simulink model "task_simulation_wo_atan_wo_saturation"  (R2025b)
settings: Solver=VariableStepAuto  StartTime=0.0  StopTime=20  FixedStep=0.001  RelTol=1e-3
InitFcn:
  | prepare_parameters
undefined symbols (not defined in the file): I_max_val, J_1_val, J_2_val, k_E_val, k_M_val, k_t_val, L_val, R_val, U_max_val
libraries: simulink_extras x5, slpidlib x2, embmathops x1
settings Model: Creator=10120  LastModifiedBy=10120

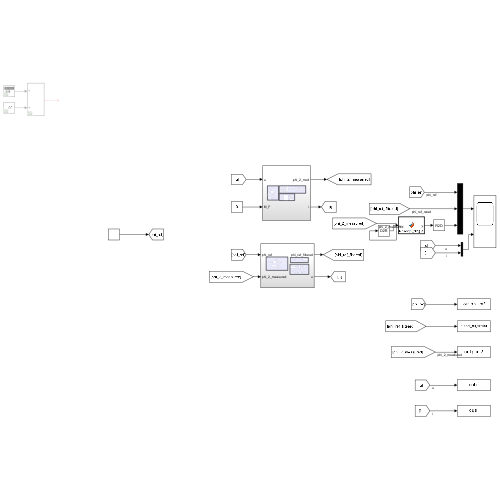
[thumbnail: Simulink's stored preview of the top-level diagram]
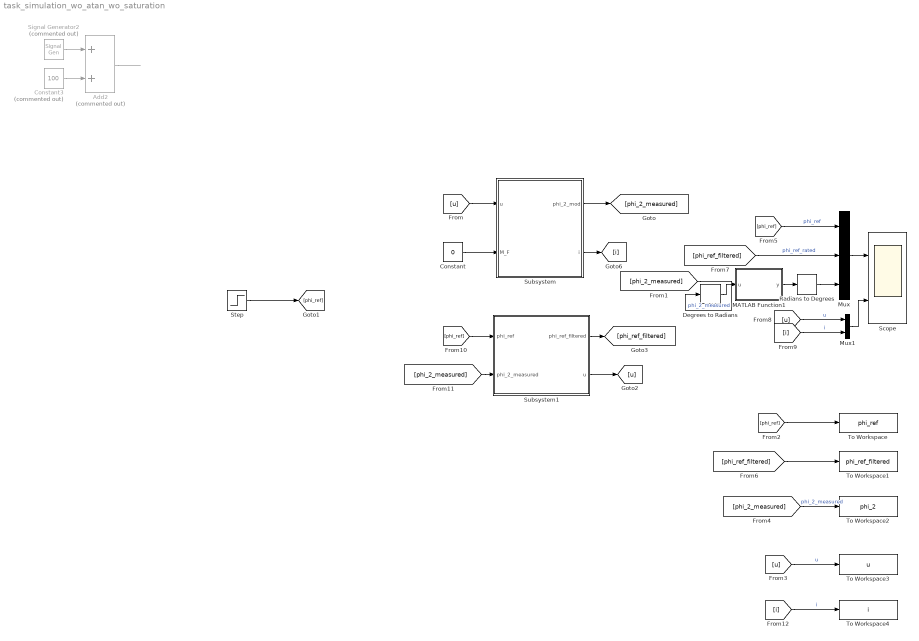
== system task_simulation_wo_atan_wo_saturation ==
  Add2 : Sum  Commented=on
  Constant : Constant  Value=0
  Constant3 : Constant  Commented=on  Value=100
  Degrees to Radians : simulink_extras/Transformations/Degrees to Radians
  MATLAB Function1 : MATLAB Function  TreatAsAtomicUnit=on
  Mux : Mux  Inputs=3
  Mux1 : Mux  Inputs=2
  Radians to Degrees : simulink_extras/Transformations/Radians to Degrees
  Scope : Scope  NumInputPorts=2
      settings: ActiveDisplayYMinimum=-44.999984027825569  ActiveDisplayYMaximum=404.99985625043018
  Signal Generator2 : SignalGenerator  Commented=on  Amplitude=100  Frequency=0.1  Units=rad/sec
  Step : Step  Time=0.1  After=200  SampleTime=0
  Subsystem : Subsystem
  Subsystem1 : Subsystem
  To Workspace : ToWorkspace  VariableName=phi_ref  SaveFormat=Structure With Time  SampleTime=-1
  To Workspace1 : ToWorkspace  VariableName=phi_ref_filtered  SaveFormat=Structure With Time  SampleTime=-1
  To Workspace2 : ToWorkspace  VariableName=phi_2  SaveFormat=Structure With Time  SampleTime=-1
  To Workspace3 : ToWorkspace  VariableName=u  SaveFormat=Structure With Time  SampleTime=-1
  To Workspace4 : ToWorkspace  VariableName=i  SaveFormat=Structure With Time  SampleTime=-1
  wires:
  Constant/1 -> Subsystem/2(M_F)
  [u] -> Subsystem/1(u)
  Subsystem/1(phi_2_mod) -> [phi_2_measured]
  Step/1 -> [phi_ref]
  Add2/1 -> ?
  Constant3/1 -> Add2/2
  Signal Generator2/1 -> Add2/1
  Mux/1 -> Scope/1
  [phi_ref] -> Mux/1  "phi_ref"
  [phi_ref_filtered] -> Mux/2  "phi_ref_rated"
  Subsystem/2(i) -> [i]
  [phi_ref] -> Subsystem1/1(phi_ref)
  [phi_2_measured] -> Subsystem1/2(phi_2_measured)
  Subsystem1/2(u) -> [u]
  Subsystem1/1(phi_ref_filtered) -> [phi_ref_filtered]
  Mux1/1 -> Scope/2
  [u] -> Mux1/1  "u"
  [i] -> Mux1/2  "i"
  [phi_ref] -> To Workspace/1
  [phi_ref_filtered] -> To Workspace1/1
  [phi_2_measured] -> To Workspace2/1  "phi_2_measured"
  [u] -> To Workspace3/1  "u"
  [i] -> To Workspace4/1  "i"
  Degrees to Radians/1 -> MATLAB Function1/1(u)
  MATLAB Function1/1(y) -> Radians to Degrees/1
  Radians to Degrees/1 -> Mux/3
  [phi_2_measured] -> Degrees to Radians/1  "phi_2_measured"

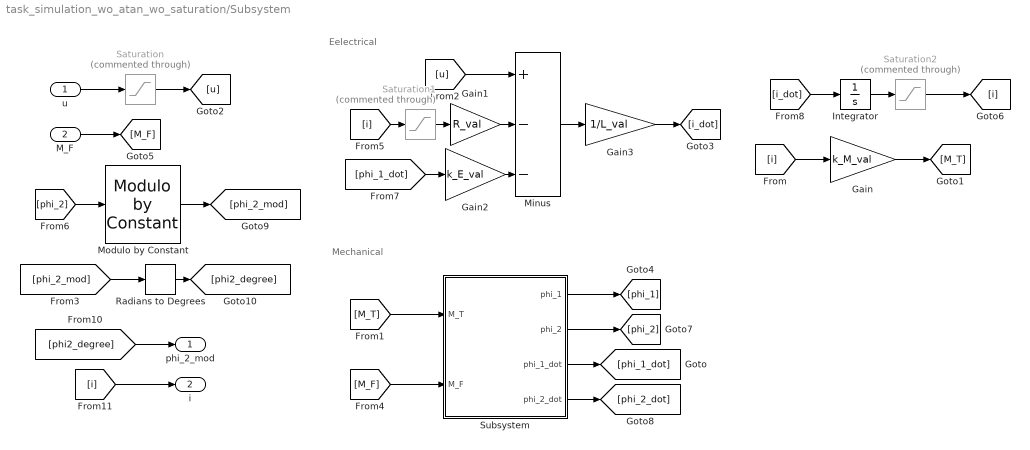
== system task_simulation_wo_atan_wo_saturation/Subsystem ==
  note: Mechanical
  note: Eelectrical
  u : Inport
  M_F : Inport  Port=2
  Gain : Gain  Gain=k_M_val
  Gain1 : Gain  Gain=R_val
  Gain2 : Gain  Gain=k_E_val
  Gain3 : Gain  Gain=1/L_val
  Integrator : Integrator
  Minus : Sum  Inputs=+--
  Modulo by Constant : embmathops/Modulo by Constant  Denominator=2*pi  SimulateUsing=Code generation
      settings: LibrarySourceBlock=embeddedMathLib/Modulo by Constant
  Radians to Degrees : simulink_extras/Transformations/Radians to Degrees
  Saturation : Saturate  Commented=through  UpperLimit=U_max_val  LowerLimit=-U_max_val
  Saturation1 : Saturate  Commented=through  UpperLimit=I_max_val  LowerLimit=-I_max_val
  Saturation2 : Saturate  Commented=through  UpperLimit=I_max_val  LowerLimit=-I_max_val
  Subsystem : Subsystem
  phi_2_mod : Outport
  i : Outport  Port=2
  wires:
  [i] -> Gain/1
  Gain/1 -> [M_T]
  [M_T] -> Subsystem/1(M_T)
  u/1 -> Saturation/1
  Gain3/1 -> [i_dot]
  [u] -> Minus/1
  Gain1/1 -> Minus/2
  [i] -> Saturation1/1
  Subsystem/1(phi_1) -> [phi_1]
  Gain2/1 -> Minus/3
  [phi_1_dot] -> Gain2/1
  Minus/1 -> Gain3/1
  [i_dot] -> Integrator/1
  Integrator/1 -> Saturation2/1
  Subsystem/3(phi_1_dot) -> [phi_1_dot]
  [phi2_degree] -> phi_2_mod/1
  M_F/1 -> [M_F]
  [M_F] -> Subsystem/2(M_F)
  Subsystem/2(phi_2) -> [phi_2]
  Subsystem/4(phi_2_dot) -> [phi_2_dot]
  [phi_2] -> Modulo by Constant/1
  Modulo by Constant/1 -> [phi_2_mod]
  Saturation/1 -> [u]
  Saturation1/1 -> Gain1/1
  Saturation2/1 -> [i]
  [i] -> i/1
  [phi_2_mod] -> Radians to Degrees/1
  Radians to Degrees/1 -> [phi2_degree]

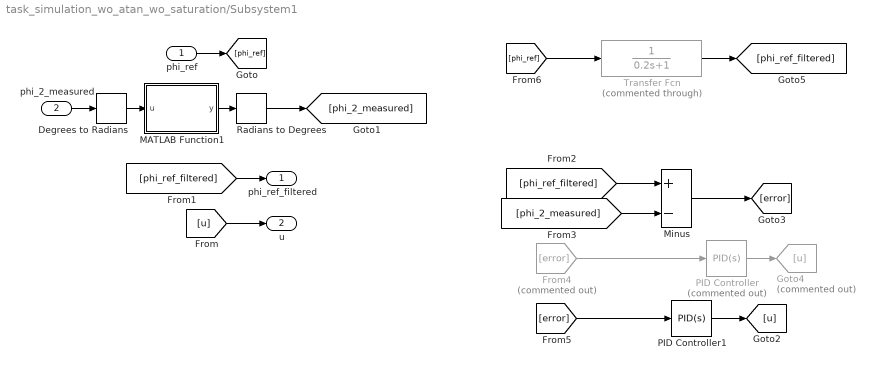
== system task_simulation_wo_atan_wo_saturation/Subsystem1 ==
  phi_ref : Inport
  phi_2_measured : Inport  Port=2
  Degrees to Radians : simulink_extras/Transformations/Degrees to Radians
  From4 : From  Commented=on  GotoTag=error
  Goto4 : Goto  Commented=on  GotoTag=u
  MATLAB Function1 : MATLAB Function  TreatAsAtomicUnit=on
  Minus : Sum  Inputs=+-
  PID Controller : slpidlib/PID Controller  Commented=on  Controller=PID  Form=Parallel  TimeDomain=Continuous-time  UseExternalTs=off  SampleTime=-1  IntegratorMethod=Forward Euler  FilterMethod=Forward Euler  ControllerParametersSource=internal  P=0.02  I=0  UseKiTs=off  D=0.5/360  UseExternalDerivativeSource=off  N=1  UseFilter=on  TunerSelectOption=Transfer Function Based (PID Tuner App)  InitialConditionSource=internal  InitialConditionForIntegrator=0  InitialConditionForFilter=0  DifferentiatorICPrevScaledInput=0  ExternalReset=none  TrackingMode=off  Kt=1  LimitOutput=on  SatLimitsSource=internal  UpperSaturationLimit=U_max_val  LowerSaturationLimit=-U_max_val  LinearizeAsGain=on  AntiWindupMode=clamping  Kb=1  LimitIntegrator=off  UpperIntegratorSaturationLimit=inf  LowerIntegratorSaturationLimit=-inf  POutMin=[]  POutMax=[]  IOutMin=[]  IOutMax=[]  DOutMin=[]  DOutMax=[]  NOutMin=[]  NOutMax=[]  SumOutMin=[]  SumOutMax=[]  SaturationOutMin=[]  SaturationOutMax=[]  PParamMin=[]  PParamMax=[]  IParamMin=[]  IParamMax=[]  DParamMin=[]  DParamMax=[]  NParamMin=[]  NParamMax=[]  KbParamMin=[]  KbParamMax=[]  KtParamMin=[]  KtParamMax=[]  KbOutMin=[]  KbOutMax=[]  KtOutMin=[]  KtOutMax=[]  IntegratorOutMin=[]  IntegratorOutMax=[]  FilterOutMin=[]  FilterOutMax=[]  SumI1OutMin=[]  SumI1OutMax=[]  SumI2OutMin=[]  SumI2OutMax=[]  SumI3OutMin=[]  SumI3OutMax=[]  SumI4OutMin=[]  SumI4OutMax=[]  SumDOutMin=[]  SumDOutMax=[]  DifferentiatorOutMin=[]  DifferentiatorOutMax=[]  FilterDiffOutCoefMin=[]  FilterDiffOutCoefMax=[]  ReciprocalOutMin=[]  ReciprocalOutMax=[]  SumDenOutMin=[]  SumDenOutMax=[]  SumNumOutMin=[]  SumNumOutMax=[]  DivideOutMin=[]  DivideOutMax=[]  UdiffTsProdOutMin=[]  UdiffTsProdOutMax=[]  NTsProdOutMin=[]  NTsProdOutMax=[]  UintegralTsProdOutMin=[]  UintegralTsProdOutMax=[]  UngainTsProdOutMin=[]  UngainTsProdOutMax=[]  ClampingZeroOutDataTypeStr=Inherit: Inherit via back propagation  ClampingZeroOutMin=[]  ClampingZeroOutMax=[]  FilterDenConstantOutDataTypeStr=Inherit: Inherit via back propagation  FilterDenConstantOutMin=[]  FilterDenConstantOutMax=[]  PCopyOutDataTypeStr=Inherit: Inherit via back propagation  PCopyOutMin=[]  PCopyOutMax=[]  NCopyOutDataTypeStr=Inherit: Inherit via back propagation  NCopyOutMin=[]  NCopyOutMax=[]  IntegratorContinuousStateAttributes=''  IntegratorStateMustResolveToSignalObject=off  IntegratorRTWStateStorageClass=Auto  FilterContinuousStateAttributes=''  FilterStateMustResolveToSignalObject=off  FilterRTWStateStorageClass=Auto  ParallelPVariant=InternalParameters  IdealPVariant=Disabled  IVariant=InternalParameters  DVariant=InternalParameters  IntegratorVariant=Continuous  SatVariant=Enabled  AWVariant=ContClampingParallel  PCopyVariant=Disabled  TRVariant=Disabled  FdbkBlocksVariant=Forward  IdealPFdbkVariant=Disabled  SatFdbkVariant=Disabled  DerivativeFilterVariant=ContFilter  NVariant=InternalParameters  NCopyVariant=Disabled  FilterICVariant=InternalICsFilter  IntegratorICVariant=InternalICs  ExternalResetVariant=Disabled  TRSumVariant=Passthrough  SumFdbkVariant=Disabled  SumVariant=Sum_PID  TsampFilterVariant=InternalTs  TsampNgainVariant=Passthrough  TsampIntegralVariant=Disabled_SignalSpec  ExternalSaturationOutDataTypeStr=Inherit: Same as second input  DerivativeSourceVariant=ErrorSignal  PreIntVariant=InternalPreInt
  PID Controller1 : slpidlib/PID Controller  Controller=PID  Form=Parallel  TimeDomain=Continuous-time  UseExternalTs=off  SampleTime=-1  IntegratorMethod=Forward Euler  FilterMethod=Forward Euler  ControllerParametersSource=internal  P=1  I=0  UseKiTs=off  D=0  UseExternalDerivativeSource=off  N=1  UseFilter=on  TunerSelectOption=Transfer Function Based (PID Tuner App)  InitialConditionSource=internal  InitialConditionForIntegrator=0  InitialConditionForFilter=0  DifferentiatorICPrevScaledInput=0  ExternalReset=none  TrackingMode=off  Kt=1  LimitOutput=off  SatLimitsSource=internal  UpperSaturationLimit=U_max_val  LowerSaturationLimit=-U_max_val  LinearizeAsGain=on  AntiWindupMode=clamping  Kb=1  LimitIntegrator=off  UpperIntegratorSaturationLimit=inf  LowerIntegratorSaturationLimit=-inf  POutMin=[]  POutMax=[]  IOutMin=[]  IOutMax=[]  DOutMin=[]  DOutMax=[]  NOutMin=[]  NOutMax=[]  SumOutMin=[]  SumOutMax=[]  SaturationOutMin=[]  SaturationOutMax=[]  PParamMin=[]  PParamMax=[]  IParamMin=[]  IParamMax=[]  DParamMin=[]  DParamMax=[]  NParamMin=[]  NParamMax=[]  KbParamMin=[]  KbParamMax=[]  KtParamMin=[]  KtParamMax=[]  KbOutMin=[]  KbOutMax=[]  KtOutMin=[]  KtOutMax=[]  IntegratorOutMin=[]  IntegratorOutMax=[]  FilterOutMin=[]  FilterOutMax=[]  SumI1OutMin=[]  SumI1OutMax=[]  SumI2OutMin=[]  SumI2OutMax=[]  SumI3OutMin=[]  SumI3OutMax=[]  SumI4OutMin=[]  SumI4OutMax=[]  SumDOutMin=[]  SumDOutMax=[]  DifferentiatorOutMin=[]  DifferentiatorOutMax=[]  FilterDiffOutCoefMin=[]  FilterDiffOutCoefMax=[]  ReciprocalOutMin=[]  ReciprocalOutMax=[]  SumDenOutMin=[]  SumDenOutMax=[]  SumNumOutMin=[]  SumNumOutMax=[]  DivideOutMin=[]  DivideOutMax=[]  UdiffTsProdOutMin=[]  UdiffTsProdOutMax=[]  NTsProdOutMin=[]  NTsProdOutMax=[]  UintegralTsProdOutMin=[]  UintegralTsProdOutMax=[]  UngainTsProdOutMin=[]  UngainTsProdOutMax=[]  ClampingZeroOutDataTypeStr=Inherit: Inherit via back propagation  ClampingZeroOutMin=[]  ClampingZeroOutMax=[]  FilterDenConstantOutDataTypeStr=Inherit: Inherit via back propagation  FilterDenConstantOutMin=[]  FilterDenConstantOutMax=[]  PCopyOutDataTypeStr=Inherit: Inherit via back propagation  PCopyOutMin=[]  PCopyOutMax=[]  NCopyOutDataTypeStr=Inherit: Inherit via back propagation  NCopyOutMin=[]  NCopyOutMax=[]  IntegratorContinuousStateAttributes=''  IntegratorStateMustResolveToSignalObject=off  IntegratorRTWStateStorageClass=Auto  FilterContinuousStateAttributes=''  FilterStateMustResolveToSignalObject=off  FilterRTWStateStorageClass=Auto  ParallelPVariant=InternalParameters  IdealPVariant=Disabled  IVariant=InternalParameters  DVariant=InternalParameters  IntegratorVariant=Continuous  SatVariant=Disabled  AWVariant=Passthrough  PCopyVariant=Disabled  TRVariant=Disabled  FdbkBlocksVariant=Forward  IdealPFdbkVariant=Disabled  SatFdbkVariant=Disabled  DerivativeFilterVariant=ContFilter  NVariant=InternalParameters  NCopyVariant=Disabled  FilterICVariant=InternalICsFilter  IntegratorICVariant=InternalICs  ExternalResetVariant=Disabled  TRSumVariant=Passthrough  SumFdbkVariant=Disabled  SumVariant=Sum_PID  TsampFilterVariant=InternalTs  TsampNgainVariant=Passthrough  TsampIntegralVariant=Disabled_SignalSpec  ExternalSaturationOutDataTypeStr=Inherit: Same as second input  DerivativeSourceVariant=ErrorSignal  PreIntVariant=InternalPreInt
  Radians to Degrees : simulink_extras/Transformations/Radians to Degrees
  Transfer Fcn : TransferFcn  Commented=through  Denominator=[0.2 1]
  phi_ref_filtered : Outport
  u : Outport  Port=2
  wires:
  Minus/1 -> [error]
  PID Controller/1 -> Goto4/1
  From4/1 -> PID Controller/1
  Transfer Fcn/1 -> [phi_ref_filtered]
  [phi_2_measured] -> Minus/2
  [phi_ref] -> Transfer Fcn/1
  [phi_ref_filtered] -> Minus/1
  phi_ref/1 -> [phi_ref]
  phi_2_measured/1 -> Degrees to Radians/1
  [phi_ref_filtered] -> phi_ref_filtered/1
  [u] -> u/1
  PID Controller1/1 -> [u]
  [error] -> PID Controller1/1
  Degrees to Radians/1 -> MATLAB Function1/1(u)
  MATLAB Function1/1(y) -> Radians to Degrees/1
  Radians to Degrees/1 -> [phi_2_measured]

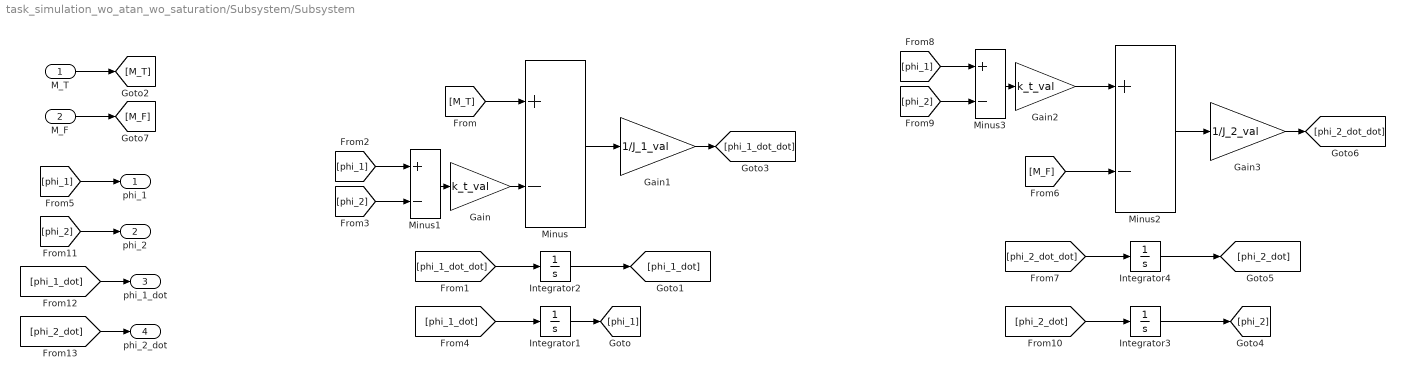
== system task_simulation_wo_atan_wo_saturation/Subsystem/Subsystem ==
  M_T : Inport
  M_F : Inport  Port=2
  Gain : Gain  Gain=k_t_val
  Gain1 : Gain  Gain=1/J_1_val
  Gain2 : Gain  Gain=k_t_val
  Gain3 : Gain  Gain=1/J_2_val
  Integrator{1..4} (4 alike) : Integrator
  Minus{,1..3} (4 alike) : Sum  Inputs=+-
  phi_1 : Outport
  phi_2 : Outport  Port=2
  phi_1_dot : Outport  Port=3
  phi_2_dot : Outport  Port=4
  wires:
  [phi_1_dot] -> Integrator1/1
  Integrator1/1 -> [phi_1]
  Integrator2/1 -> [phi_1_dot]
  [phi_1_dot_dot] -> Integrator2/1
  M_T/1 -> [M_T]
  [M_T] -> Minus/1
  Minus1/1 -> Gain/1
  [phi_1] -> Minus1/1
  [phi_2] -> Minus1/2
  Gain/1 -> Minus/2
  Minus/1 -> Gain1/1
  Gain1/1 -> [phi_1_dot_dot]
  [phi_1] -> phi_1/1
  [phi_2_dot] -> Integrator3/1
  Integrator3/1 -> [phi_2]
  [phi_2_dot_dot] -> Integrator4/1
  Minus2/1 -> Gain3/1
  [phi_2] -> Minus3/2
  Integrator4/1 -> [phi_2_dot]
  Minus3/1 -> Gain2/1
  Gain3/1 -> [phi_2_dot_dot]
  [phi_1] -> Minus3/1
  Gain2/1 -> Minus2/1
  M_F/1 -> [M_F]
  [M_F] -> Minus2/2
  [phi_2] -> phi_2/1
  [phi_1_dot] -> phi_1_dot/1
  [phi_2_dot] -> phi_2_dot/1

== matlab function task_simulation_wo_atan_wo_saturation/Subsystem1/MATLAB Function1 ==
  data: u input; y output
function y = unwrap_angle(u)
%#codegen
y = unwrap(u);
end

== matlab function task_simulation_wo_atan_wo_saturation/MATLAB Function1 ==
  data: u input; y output
function y = unwrap_angle(u)
%#codegen
y = unwrap(u);
end
